simulink model "MaxPilot"  (R2026a)
settings: Solver=VariableStepAuto  StopTime=30
settings Model: Creator=max  LastModifiedBy=Owner

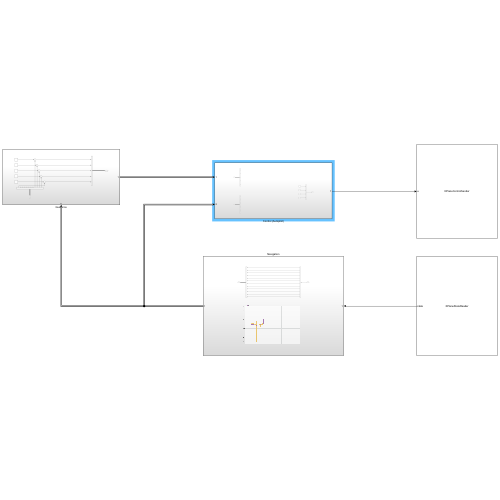
[thumbnail: Simulink's stored preview of the top-level diagram]
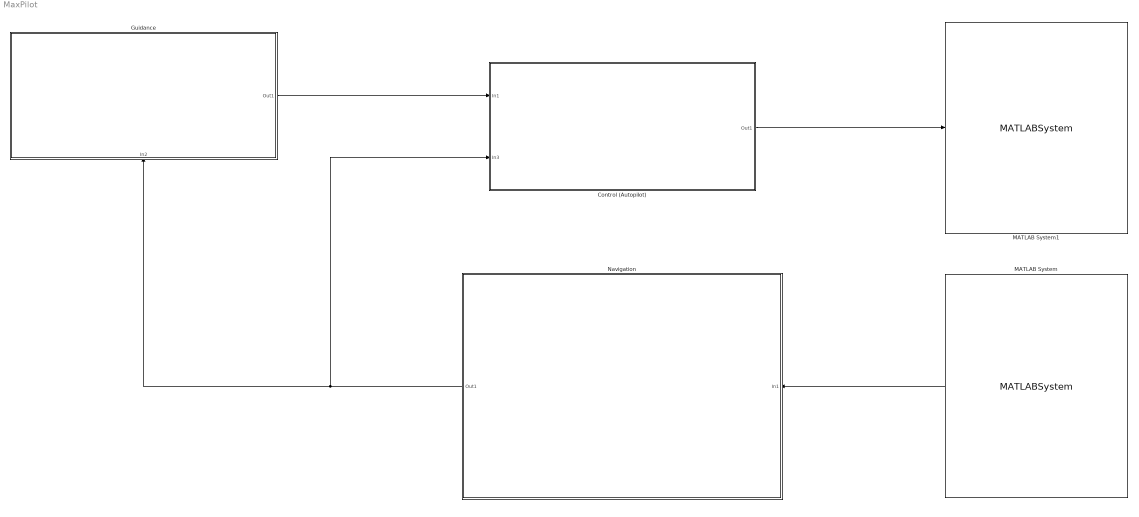
== system MaxPilot ==
  Control (Autopilot) : Subsystem
  Guidance : Subsystem
      settings: PortSchema="{\"entries\":[{\"content\":{\"sides\":[{\"content\":{},\"type\":\"ConnectorPlacement.EquallySpacedRectSide\",\"uuid\":\"e11f845c-727a-4623-8abb-a86b842d9894\"},{\"content\":{\"connectorIds\":[\"Out1\"],\"side\":\"RIGHT\"},\"type\":\"ConnectorPlacement.EquallySpacedRectSide\",\"uuid\":\"0ead8184-70d2-4c1b-98dc-64e560e2a903\"},{\"content\":{\"side\":\"TOP\"},\"type\":\"ConnectorPlacement.EquallySpacedRectSide\",\"uuid\":\"faab937e-1283-4214-83c9-3a230b74f371\"},{\"content\":{\"connectorIds\":[\"In1\"],\"side\":\"BOTTOM\"},\"type\":\"ConnectorPlacement.EquallySpacedRectSide\",\"uuid\":\"89b0e162-5b11-45eb-99f5-a61c863778c0\"}]},\"type\":\"ConnectorPlacement.EquallySpacedConnector\",\"uuid\":\"efd43e26-ed77-40df-bb71-45bc413bd349\"}],\"packageUris\":[\"http://schema.mathworks.com/mf0/Connector/R2020b\"],\"version\":\"1.0\"}"
  MATLAB System : MATLABSystem  System=XPlaneStateReader  SimulateUsing=Interpreted execution
      mask Type: XPlaneStateReader
  MATLAB System1 : MATLABSystem  System=XPlaneControlSender  SimulateUsing=Interpreted execution
      mask Type: XPlaneControlSender
  Navigation : Subsystem
  wires:
  Guidance/1(Out1) -> Control (Autopilot)/1(In1)
  MATLAB System/1 -> Navigation/1(In1)
  Navigation/1(Out1) -> Control (Autopilot)/2(In3), Guidance/1(In2)
  Control (Autopilot)/1(Out1) -> MATLAB System1/1

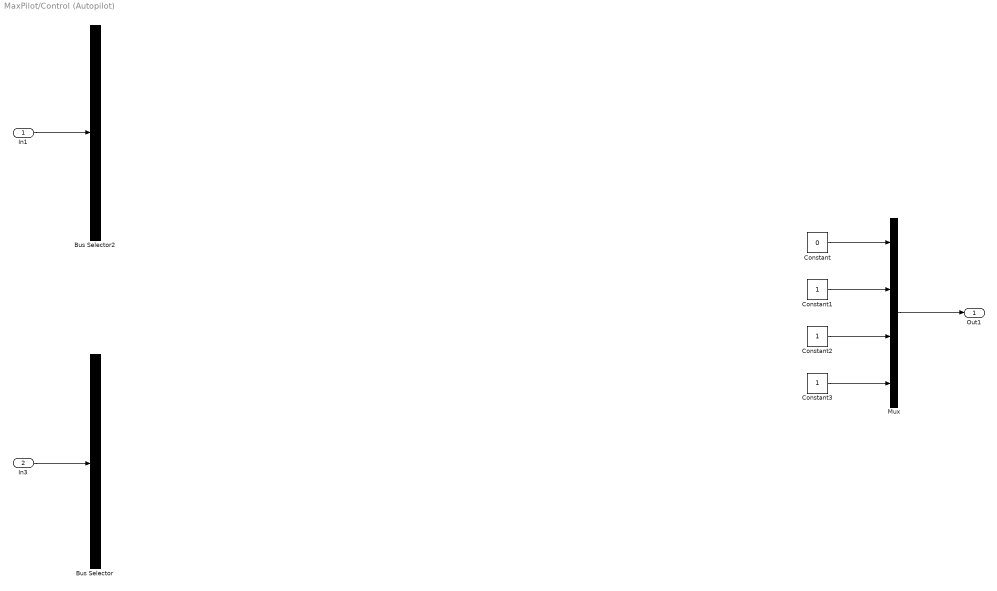
== system MaxPilot/Control (Autopilot) ==
  In1 : Inport
  In3 : Inport  Port=2
  Bus Selector : BusSelector  OutputSignals=u,v,w,p,q,r,phi,theta,psi,North,East,alt
  Bus Selector2 : BusSelector  OutputSignals=psi_e,North_e,East_e,alt_e,u_e
  Constant : Constant  Value=0
  Constant1 : Constant
  Constant2 : Constant
  Constant3 : Constant
  Mux : Mux
  Out1 : Outport
  wires:
  In3/1 -> Bus Selector/1
  In1/1 -> Bus Selector2/1
  Mux/1 -> Out1/1
  Constant/1 -> Mux/1
  Constant1/1 -> Mux/2
  Constant2/1 -> Mux/3
  Constant3/1 -> Mux/4

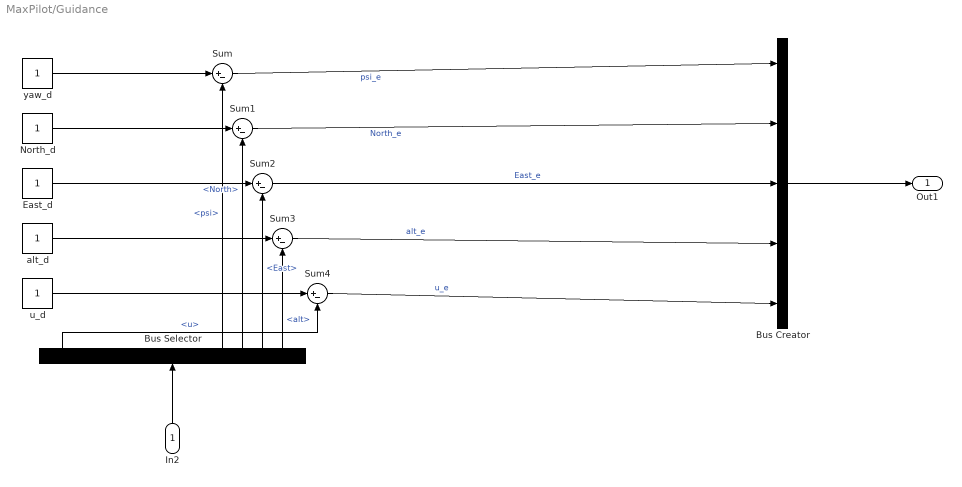
== system MaxPilot/Guidance ==
  In2 : Inport
  Bus Creator : BusCreator  Inputs=5
  Bus Selector : BusSelector  OutputSignals=u,v,w,p,q,r,phi,theta,psi,North,East,alt
  East_d : Constant
  North_d : Constant
  Sum{,1..4} (5 alike) : Sum  Inputs=|+-
  alt_d : Constant
  u_d : Constant
  yaw_d : Constant
  Out1 : Outport
  wires:
  In2/1 -> Bus Selector/1
  Bus Creator/1 -> Out1/1
  Bus Selector/12 -> Sum3/2  "<alt>"
  Bus Selector/11 -> Sum2/2  "<East>"
  Bus Selector/10 -> Sum1/2  "<North>"
  Bus Selector/9 -> Sum/2  "<psi>"
  alt_d/1 -> Sum3/1
  East_d/1 -> Sum2/1
  North_d/1 -> Sum1/1
  yaw_d/1 -> Sum/1
  Sum/1 -> Bus Creator/1  "psi_e"
  Sum1/1 -> Bus Creator/2  "North_e"
  Sum2/1 -> Bus Creator/3  "East_e"
  Sum3/1 -> Bus Creator/4  "alt_e"
  Bus Selector/1 -> Sum4/2  "<u>"
  u_d/1 -> Sum4/1
  Sum4/1 -> Bus Creator/5  "u_e"

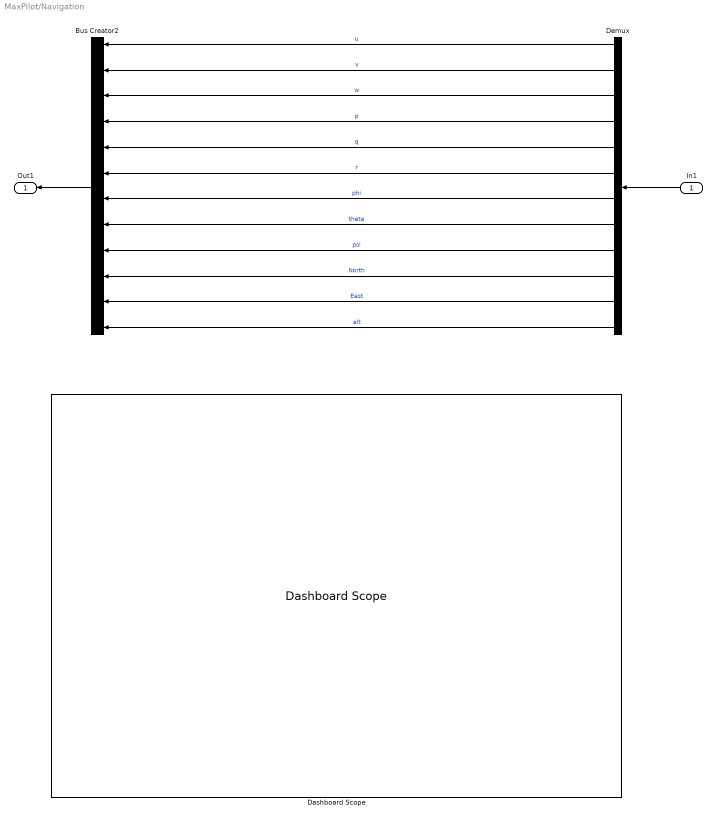
== system MaxPilot/Navigation ==
  In1 : Inport
  Bus Creator2 : BusCreator  Inputs=12
  Dashboard Scope : DashboardScope  FontColor=[0.0, 0.0, 0.0]
  Demux : Demux  Outputs=12
  Out1 : Outport
  wires:
  Demux/2 -> Bus Creator2/2  "v"
  Demux/1 -> Bus Creator2/1  "u"
  Demux/3 -> Bus Creator2/3  "w"
  Demux/4 -> Bus Creator2/4  "p"
  Demux/5 -> Bus Creator2/5  "q"
  Demux/6 -> Bus Creator2/6  "r"
  Demux/7 -> Bus Creator2/7  "phi"
  Demux/8 -> Bus Creator2/8  "theta"
  Demux/9 -> Bus Creator2/9  "psi"
  Demux/10 -> Bus Creator2/10  "North"
  Demux/11 -> Bus Creator2/11  "East"
  In1/1 -> Demux/1
  Demux/12 -> Bus Creator2/12  "alt"
  Bus Creator2/1 -> Out1/1
